simulink model "Vicon_04Sep2012_2Agents"  (Simulink 7.7)
settings: Solver=ode4  StartTime=0.0  StopTime=inf  FixedStep=sample_time  RelTol=1e-3
PreLoadFcn:
  | addpath([cd filesep 'MATLAB_vicon']);
  | addpath([cd filesep 'MATLAB_vicon\Microsoft.VC90.CRT']);
InitFcn:
  | sample_time=0.01;
libraries: simulink x6
settings Model: Creator=ttcl3  LastModifiedBy=Soon Hooi Chiew
settings SolverCC: MaxConsecutiveMinStep=auto
settings DebuggingCC: MultiTaskRateTransMsg=warning

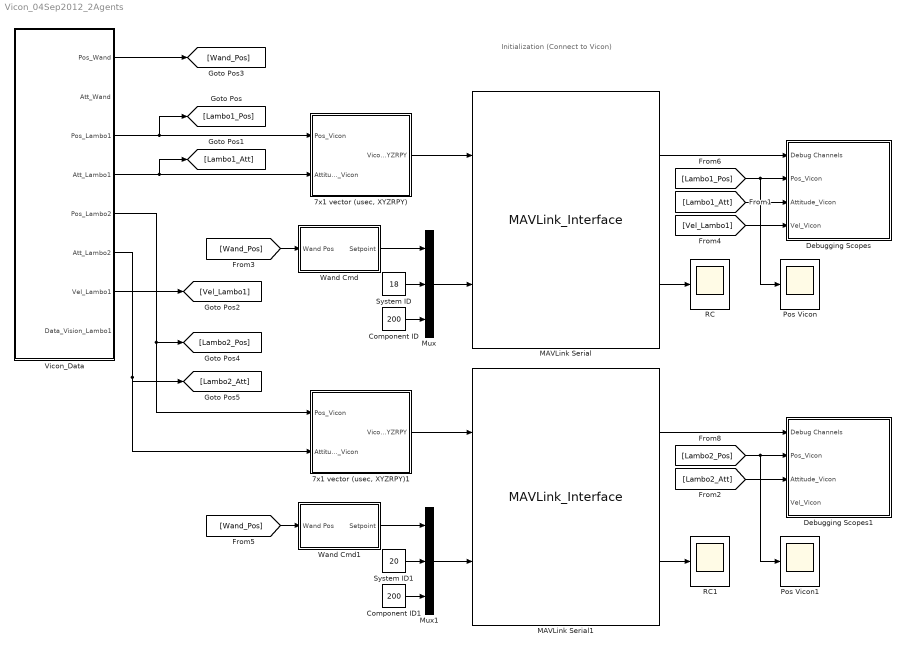
== system Vicon_04Sep2012_2Agents ==
  note: Initialization
      | (Connect to Vicon)
  "7x1 vector (usec, XYZRPY)" : Subsystem
  "7x1 vector (usec, XYZRPY)1" : Subsystem
  Component ID : Constant  Value=200  SampleTime=sample_time
  Component ID1 : Constant  Value=200  SampleTime=sample_time
  Debugging Scopes : Subsystem
  Debugging Scopes1 : Subsystem
  MAVLink Serial : S-Function  FunctionName=MAVLink_Interface  Parameters=COM_Port,Baud_Rate,MSG_INPUT,MSG_OUTPUT  EnableBusSupport=off  mask{COM_Port='COM8', Baud_Rate=57600, HEART_BEAT=off, ATTITUDE_OUT=on, RAW_IMU=off, POSITION_OUT=off, VFR_HUD=off, RC_SCALED=on, SERVO_OUT_RAW=off, VICON_XYZ_RPY_Output=off, SET_MODE=off, DATA_STREAM=off, ATTITUDE_COMMAND=off, ATTITUDE_IN=off, GPS_RAW_IN=off, VFR_HUD_IN=off, VICON_XYZ_RPY=on, VICON_VEL=off, POSITION_DESIRED=on}
      mask prompts: COM_Port "COM Port"; Baud_Rate "Baud Rate"; HEART_BEAT "HEART BEAT"; ATTITUDE_OUT "ATTITUDE"; RAW_IMU "RAW IMU"; POSITION_OUT "GLOBAL POSITION"; VFR_HUD "VFR HUD"; RC_SCALED "RC CHANNELS SCALED"; SERVO_OUT_RAW "SERVO OUTPUT RAW"; VICON_XYZ_RPY_Output "VICON Output"; SET_MODE "SET MODE"; DATA_STREAM "REQUEST DATA STREAM"; ATTITUDE_COMMAND "ATTITUDE COMMAND"; ATTITUDE_IN "ATTITUDE (HIL)"; GPS_RAW_IN "GPS RAW (HIL)"; VFR_HUD_IN "AIRSPEED (HIL)"; VICON_XYZ_RPY "VICON POSITION"; VICON_VEL "VICON SPEED"; POSITION_DESIRED "Position Desired"
      mask init:
      | MSG_ID_NUM_INPUT = [uint8(11) uint8(66) uint8(59) uint8(30) uint8(32) uint8(73) uint8(104) uint8(103) uint8(50)];
      | MSG_ID_NAME_INPUT = [SET_MODE DATA_STREAM ATTITUDE_COMMAND ATTITUDE_IN GPS_RAW_IN VFR_HUD_IN VICON_XYZ_RPY VICON_VEL POSITION_DESIRED];
      | 
      | MSG_ID_NUM_OUTPUT = [uint8(0) uint8(30) uint8(27) uint8(73) uint8(74) uint8(34) uint8(37) uint8(104)];
      | MSG_ID_NAME_OUTPUT = [HEART_BEAT ATTITUDE_OUT RAW_IMU VFR_HUD POSITION_OUT RC_SCALED SERVO_OUT_RAW VICON_XYZ_RPY_Output];
      | 
      | idx_input = find(MSG_ID_NAME_INPUT);
      | MSG_INPUT = MSG_ID_NUM_INPUT(idx_input);
      | 
      | idx_output = find(MSG_ID_NAME_OUTPUT);
      | MSG_OUTPUT = MSG_ID_NUM_OUTPUT(idx_output);
      mask TabNameString: Setting,Setting,Output Message,Output Message,Output Message,Output Message,Output Message,Output Message,Output Message,Output Message,Input Message,Input Message,Input Message,Input Message,Input Message,Input Message,Input Message,Input Message,Input Message
      mask Display:
      | %Label block
      | fprintf('MAVLink Serial\n%s\n%dbps', COM_Port,  Baud_Rate)
      | 
      | %Label input ports
      | 
      | in = 1;
      | if (SET_MODE == 1)
      |     port_label('input', in, 'SET MODE');
      |     in = in + 1;
      | end
      | if (DATA_STREAM == 1)
      |     port_label('input', in, 'REQUEST DATA STREAM');
      |     in = in + 1;
      | end
      | if (ATTITUDE_COMMAND == 1)
      |     port_label('input', in, 'ATTITUDE COMMAND');
      |     in = in + 1;
      | end
      | if (ATTITUDE_IN == 1)
      |     port_label('input', in, 'ATTITUDE (HIL)');
      |     in = in + 1;
      | end
      | if (GPS_RAW_IN == 1)
      |     port_label('input', in, 'GPS RAW (HIL)');
      |     in = in + 1;
      | end
      | if (VFR_HUD_IN == 1)
      |     port_label('input', in, 'AIRSPEED (HIL)');
      |     in = in + 1;
      | end
      | if (VICON_XYZ_RPY == 1)
      |     port_label('input', in, 'VICON XYZ RPY');
      |     in = in + 1;
      | end
      | if (VICON_VEL == 1)
      |     port_label('input', in, 'VICON_VEL');
      |     in = in + 1;
      | end
      | 
      | if (POSITION_DESIRED == 1)
      |     port_label('input', in, 'POSITION_DESIRED');
      |     in = in + 1;
      | end
      | 
      | %Label output ports
      | 
      | out = 1;
      | if (HEART_BEAT == 1)
      |     port_label('output', out, 'HEART BEAT');
      |     out = out + 1;
      | end
      | if (ATTITUDE_OUT == 1)
      |     port_label('output', out, 'ATTITUDE');
      |     out = out + 1;
      | end
      | if (RAW_IMU == 1)
      |     port_label('output', out, 'RAW IMU');
      |     out = out + 1;
      | end
      | if (POSITION_OUT == 1)
      |     port_label('output', out, 'GLOBAL POSITION');
      |     out = out + 1;
      | end
      | if (VFR_HUD == 1)
      |     port_label('output', out, 'VFR HUD');
      |     out = out + 1;
      | end
      | if (RC_SCALED == 1)
      |     port_label('output', out, 'RC CHANNELS SCALED');
      |     out = out + 1;
      | end
      | if (SERVO_OUT_RAW == 1)
      |     port_label('output', out, 'SERVO OUTPUT RAW');
      |     out = out + 1;
      | end
      | % weihua, vicon output
      | if (VICON_XYZ_RPY_Output == 1)
      |     port_label('output', out, 'VICON_XYZ_RPY');
      |     out = out + 1;
      | end
  MAVLink Serial1 : S-Function  FunctionName=MAVLink_Interface  Parameters=COM_Port,Baud_Rate,MSG_INPUT,MSG_OUTPUT  EnableBusSupport=off  mask{COM_Port='COM4', Baud_Rate=57600, HEART_BEAT=off, ATTITUDE_OUT=on, RAW_IMU=off, POSITION_OUT=off, VFR_HUD=off, RC_SCALED=on, SERVO_OUT_RAW=off, VICON_XYZ_RPY_Output=off, SET_MODE=off, DATA_STREAM=off, ATTITUDE_COMMAND=off, ATTITUDE_IN=off, GPS_RAW_IN=off, VFR_HUD_IN=off, VICON_XYZ_RPY=on, VICON_VEL=off, POSITION_DESIRED=on}
      mask prompts: COM_Port "COM Port"; Baud_Rate "Baud Rate"; HEART_BEAT "HEART BEAT"; ATTITUDE_OUT "ATTITUDE"; RAW_IMU "RAW IMU"; POSITION_OUT "GLOBAL POSITION"; VFR_HUD "VFR HUD"; RC_SCALED "RC CHANNELS SCALED"; SERVO_OUT_RAW "SERVO OUTPUT RAW"; VICON_XYZ_RPY_Output "VICON Output"; SET_MODE "SET MODE"; DATA_STREAM "REQUEST DATA STREAM"; ATTITUDE_COMMAND "ATTITUDE COMMAND"; ATTITUDE_IN "ATTITUDE (HIL)"; GPS_RAW_IN "GPS RAW (HIL)"; VFR_HUD_IN "AIRSPEED (HIL)"; VICON_XYZ_RPY "VICON POSITION"; VICON_VEL "VICON SPEED"; POSITION_DESIRED "Position Desired"
      mask init: same as Vicon_04Sep2012_2Agents/MAVLink Serial
      mask TabNameString: Setting,Setting,Output Message,Output Message,Output Message,Output Message,Output Message,Output Message,Output Message,Output Message,Input Message,Input Message,Input Message,Input Message,Input Message,Input Message,Input Message,Input Message,Input Message
      mask Display:
      | %Label block
      | fprintf('MAVLink Serial\n%s\n%dbps', COM_Port,  Baud_Rate)
      | 
      | %Label input ports
      | 
      | in = 1;
      | if (SET_MODE == 1)
      |     port_label('input', in, 'SET MODE');
      |     in = in + 1;
      | end
      | if (DATA_STREAM == 1)
      |     port_label('input', in, 'REQUEST DATA STREAM');
      |     in = in + 1;
      | end
      | if (ATTITUDE_COMMAND == 1)
      |     port_label('input', in, 'ATTITUDE COMMAND');
      |     in = in + 1;
      | end
      | if (ATTITUDE_IN == 1)
      |     port_label('input', in, 'ATTITUDE (HIL)');
      |     in = in + 1;
      | end
      | if (GPS_RAW_IN == 1)
      |     port_label('input', in, 'GPS RAW (HIL)');
      |     in = in + 1;
      | end
      | if (VFR_HUD_IN == 1)
      |     port_label('input', in, 'AIRSPEED (HIL)');
      |     in = in + 1;
      | end
      | if (VICON_XYZ_RPY == 1)
      |     port_label('input', in, 'VICON XYZ RPY');
      |     in = in + 1;
      | end
      | if (VICON_VEL == 1)
      |     port_label('input', in, 'VICON_VEL');
      |     in = in + 1;
      | end
      | 
      | if (POSITION_DESIRED == 1)
      |     port_label('input', in, 'POSITION_DESIRED');
      |     in = in + 1;
      | end
      | 
      | %Label output ports
      | 
      | out = 1;
      | if (HEART_BEAT == 1)
      |     port_label('output', out, 'HEART BEAT');
      |     out = out + 1;
      | end
      | if (ATTITUDE_OUT == 1)
      |     port_label('output', out, 'ATTITUDE');
      |     out = out + 1;
      | end
      | if (RAW_IMU == 1)
      |     port_label('output', out, 'RAW IMU');
      |     out = out + 1;
      | end
      | if (POSITION_OUT == 1)
      |     port_label('output', out, 'GLOBAL POSITION');
      |     out = out + 1;
      | end
      | if (VFR_HUD == 1)
      |     port_label('output', out, 'VFR HUD');
      |     out = out + 1;
      | end
      | if (RC_SCALED == 1)
      |     port_label('output', out, 'RC CHANNELS SCALED');
      |     out = out + 1;
      | end
      | if (SERVO_OUT_RAW == 1)
      |     port_label('output', out, 'SERVO OUTPUT RAW');
      |     out = out + 1;
      | end
      | % weihua, vicon output
      | if (VICON_XYZ_RPY_Output == 1)
      |     port_label('output', out, 'VICON_XYZ_RPY');
      |     out = out + 1;
      | end
  Mux : Mux  Inputs=3
  Mux1 : Mux  Inputs=3
  Pos Vicon : Scope
      settings: TickLabels=on  TimeRange=30  YMin=-3  YMax=3.5  SaveName=ScopeData3  SampleInput=on
  Pos Vicon1 : Scope
      settings: TickLabels=on  TimeRange=30  YMin=-3  YMax=3.5  SaveName=ScopeData17  SampleInput=on
  RC : Scope
      settings: TickLabels=on  TimeRange=30  YMin=-1  YMax=0.1  SaveName=ScopeData2  SampleInput=on
  RC1 : Scope
      settings: TickLabels=on  TimeRange=30  YMin=-1  YMax=0.1  SaveName=ScopeData18  SampleInput=on
  System ID : Constant  Value=18  SampleTime=sample_time
  System ID1 : Constant  Value=20  SampleTime=sample_time
  Vicon_Data : Subsystem
  Wand Cmd : Subsystem
  Wand Cmd1 : Subsystem
  wires:
  MAVLink Serial/1 -> Debugging Scopes/1(Debug Channels)
  [Lambo1_Pos] -> Debugging Scopes/2(Pos_Vicon), Pos Vicon/1
  [Lambo1_Att] -> Debugging Scopes/3(Attitude_Vicon)
  "7x1 vector (usec, XYZRPY)"/1(Vicon XYZRPY) -> MAVLink Serial/1
  Vicon_Data/4(Att_Lambo1) -> [Lambo1_Att], "7x1 vector (usec, XYZRPY)"/2(Attitude_Vicon)
  Mux/1 -> MAVLink Serial/2
  System ID/1 -> Mux/2
  Component ID/1 -> Mux/3
  [Vel_Lambo1] -> Debugging Scopes/4(Vel_Vicon)
  Vicon_Data/7(Vel_Lambo1) -> [Vel_Lambo1]
  Vicon_Data/3(Pos_Lambo1) -> "7x1 vector (usec, XYZRPY)"/1(Pos_Vicon), [Lambo1_Pos]
  Wand Cmd/1(Setpoint) -> Mux/1
  [Wand_Pos] -> Wand Cmd/1(Wand Pos)
  Vicon_Data/1(Pos_Wand) -> [Wand_Pos]
  MAVLink Serial/2 -> RC/1
  MAVLink Serial1/1 -> Debugging Scopes1/1(Debug Channels)
  [Lambo2_Pos] -> Pos Vicon1/1, Debugging Scopes1/2(Pos_Vicon)
  [Lambo2_Att] -> Debugging Scopes1/3(Attitude_Vicon)
  "7x1 vector (usec, XYZRPY)1"/1(Vicon XYZRPY) -> MAVLink Serial1/1
  Mux1/1 -> MAVLink Serial1/2
  System ID1/1 -> Mux1/2
  Component ID1/1 -> Mux1/3
  Wand Cmd1/1(Setpoint) -> Mux1/1
  [Wand_Pos] -> Wand Cmd1/1(Wand Pos)
  MAVLink Serial1/2 -> RC1/1
  Vicon_Data/5(Pos_Lambo2) -> "7x1 vector (usec, XYZRPY)1"/1(Pos_Vicon), [Lambo2_Pos]
  Vicon_Data/6(Att_Lambo2) -> "7x1 vector (usec, XYZRPY)1"/2(Attitude_Vicon), [Lambo2_Att]

== system Vicon_04Sep2012_2Agents/7x1 vector (usec, XYZRPY) ==
  Pos_Vicon : Inport
  Attitude_Vicon : Inport  Port=2
  Mux1 : Mux  Inputs=3
  usec : Constant  Value=0
  Vicon XYZRPY : Outport
  wires:
  usec/1 -> Mux1/1
  Pos_Vicon/1 -> Mux1/2
  Attitude_Vicon/1 -> Mux1/3
  Mux1/1 -> Vicon XYZRPY/1

== system Vicon_04Sep2012_2Agents/7x1 vector (usec, XYZRPY)1 ==
  Pos_Vicon : Inport
  Attitude_Vicon : Inport  Port=2
  Mux1 : Mux  Inputs=3
  usec : Constant  Value=0
  Vicon XYZRPY : Outport
  wires:
  Mux1/1 -> Vicon XYZRPY/1
  Attitude_Vicon/1 -> Mux1/3
  Pos_Vicon/1 -> Mux1/2
  usec/1 -> Mux1/1

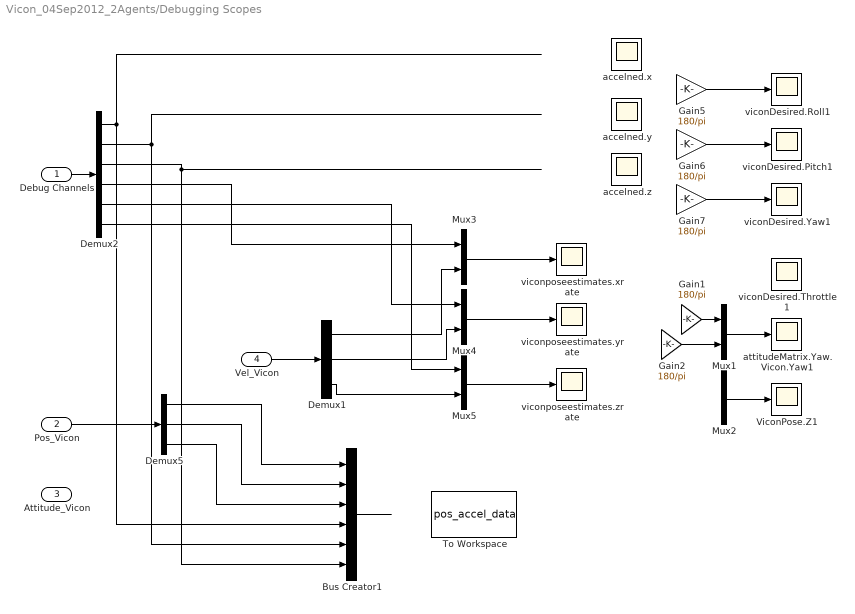
== system Vicon_04Sep2012_2Agents/Debugging Scopes ==
  Debug Channels : Inport
  Pos_Vicon : Inport  Port=2
  Attitude_Vicon : Inport  Port=3
  Vel_Vicon : Inport  Port=4
  Bus Creator1 : BusCreator  Inputs=6
  Demux1 : Demux  Outputs=3
  Demux2 : Demux  Outputs=6
  Demux5 : Demux  Outputs=3
  Gain{1..2,5..7} (5 alike) : Gain  Gain=180/pi
  Mux{1..5} (5 alike) : Mux  Inputs=2
  To Workspace : ToWorkspace  VariableName=pos_accel_data  SampleTime=sample_time  SaveFormat=Structure With Time
  ViconPose.Z1 : Scope
      settings: TickLabels=on  TimeRange=60  YMin=-0.475  YMax=-0.2  SaveName=ScopeData9  SampleInput=on
  accelned.x : Scope
      settings: TickLabels=on  TimeRange=60  YMin=-0.06  YMax=-0.0325  SampleInput=on
  accelned.y : Scope
      settings: TickLabels=on  TimeRange=25  YMin=4.12  YMax=4.34  SaveName=ScopeData13  SampleInput=on
  accelned.z : Scope
      settings: TickLabels=on  TimeRange=60  YMin=0.18  YMax=0.31  SaveName=ScopeData14  SampleInput=on
  attitudeMatrix.Yaw. Vicon.Yaw1 : Scope
      settings: TickLabels=on  TimeRange=60  YMin=-81  YMax=-72.5  SaveName=ScopeData15  SampleInput=on
  viconDesired.Pitch1 : Scope
      settings: TickLabels=on  TimeRange=25  YMin=-10.5  YMax=1  SaveName=ScopeData6  SampleInput=on
  viconDesired.Roll1 : Scope
      settings: TickLabels=on  TimeRange=60  YMax=7  SaveName=ScopeData7  SampleInput=on
  viconDesired.Throttle1 : Scope
      settings: TickLabels=on  TimeRange=60  YMin=0  YMax=0.5  SaveName=ScopeData16  SampleInput=on
  viconDesired.Yaw1 : Scope
      settings: TickLabels=on  TimeRange=60  YMin=-0.125  YMax=-0.0725  SaveName=ScopeData8  SampleInput=on
  viconposeestimates.xrate : Scope
      settings: TickLabels=on  TimeRange=60  YMin=-0.0175  YMax=0.0175  SampleInput=on
  viconposeestimates.yrate : Scope
      settings: TickLabels=on  TimeRange=60  YMin=-0.015  YMax=0.0125  SaveName=ScopeData11  SampleInput=on
  viconposeestimates.zrate : Scope
      settings: TickLabels=on  TimeRange=60  YMin=-10  YMax=60  SaveName=ScopeData12  SampleInput=on
  wires:
  Demux2/1 -> Bus Creator1/4
  Demux2/2 -> Bus Creator1/5
  Demux2/3 -> Bus Creator1/6
  Demux5/3 -> Bus Creator1/3
  Demux5/1 -> Bus Creator1/1
  Demux5/2 -> Bus Creator1/2
  Bus Creator1/1 -> ?
  Debug Channels/1 -> Demux2/1
  Pos_Vicon/1 -> Demux5/1
  Gain5/1 -> viconDesired.Roll1/1
  Gain6/1 -> viconDesired.Pitch1/1
  Gain7/1 -> viconDesired.Yaw1/1
  Mux1/1 -> attitudeMatrix.Yaw. Vicon.Yaw1/1
  Mux2/1 -> ViconPose.Z1/1
  Gain1/1 -> Mux1/1
  Gain2/1 -> Mux1/2
  Vel_Vicon/1 -> Demux1/1
  Demux2/4 -> Mux3/1
  Demux2/5 -> Mux4/1
  Demux2/6 -> Mux5/1
  Demux1/3 -> Mux5/2
  Mux3/1 -> viconposeestimates.xrate/1
  Mux4/1 -> viconposeestimates.yrate/1
  Mux5/1 -> viconposeestimates.zrate/1
  Demux1/1 -> Mux3/2
  Demux1/2 -> Mux4/2

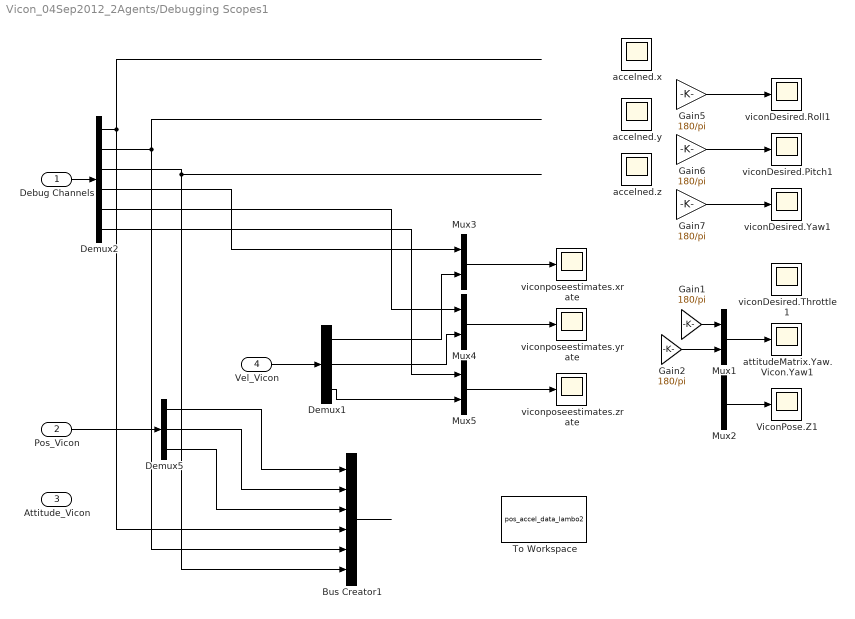
== system Vicon_04Sep2012_2Agents/Debugging Scopes1 ==
  Debug Channels : Inport
  Pos_Vicon : Inport  Port=2
  Attitude_Vicon : Inport  Port=3
  Vel_Vicon : Inport  Port=4
  Bus Creator1 : BusCreator  Inputs=6
  Demux1 : Demux  Outputs=3
  Demux2 : Demux  Outputs=6
  Demux5 : Demux  Outputs=3
  Gain{1..2,5..7} (5 alike) : Gain  Gain=180/pi
  Mux{1..5} (5 alike) : Mux  Inputs=2
  To Workspace : ToWorkspace  VariableName=pos_accel_data_lambo2  SampleTime=sample_time  SaveFormat=Structure With Time
  ViconPose.Z1 : Scope
      settings: TickLabels=on  TimeRange=60  YMin=-0.475  YMax=-0.2  SaveName=ScopeData9  SampleInput=on
  accelned.x : Scope
      settings: TickLabels=on  TimeRange=60  YMin=-0.06  YMax=-0.0325  SampleInput=on
  accelned.y : Scope
      settings: TickLabels=on  TimeRange=25  YMin=4.12  YMax=4.34  SaveName=ScopeData13  SampleInput=on
  accelned.z : Scope
      settings: TickLabels=on  TimeRange=60  YMin=0.18  YMax=0.31  SaveName=ScopeData14  SampleInput=on
  attitudeMatrix.Yaw. Vicon.Yaw1 : Scope
      settings: TickLabels=on  TimeRange=60  YMin=-81  YMax=-72.5  SaveName=ScopeData15  SampleInput=on
  viconDesired.Pitch1 : Scope
      settings: TickLabels=on  TimeRange=25  YMin=-10.5  YMax=1  SaveName=ScopeData6  SampleInput=on
  viconDesired.Roll1 : Scope
      settings: TickLabels=on  TimeRange=60  YMax=7  SaveName=ScopeData7  SampleInput=on
  viconDesired.Throttle1 : Scope
      settings: TickLabels=on  TimeRange=60  YMin=0  YMax=0.5  SaveName=ScopeData16  SampleInput=on
  viconDesired.Yaw1 : Scope
      settings: TickLabels=on  TimeRange=60  YMin=-0.125  YMax=-0.0725  SaveName=ScopeData8  SampleInput=on
  viconposeestimates.xrate : Scope
      settings: TickLabels=on  TimeRange=60  YMin=-0.0175  YMax=0.0175  SampleInput=on
  viconposeestimates.yrate : Scope
      settings: TickLabels=on  TimeRange=60  YMin=-0.015  YMax=0.0125  SaveName=ScopeData11  SampleInput=on
  viconposeestimates.zrate : Scope
      settings: TickLabels=on  TimeRange=60  YMin=-10  YMax=60  SaveName=ScopeData12  SampleInput=on
  wires:
  Demux1/2 -> Mux4/2
  Demux1/1 -> Mux3/2
  Mux5/1 -> viconposeestimates.zrate/1
  Mux4/1 -> viconposeestimates.yrate/1
  Mux3/1 -> viconposeestimates.xrate/1
  Demux1/3 -> Mux5/2
  Demux2/6 -> Mux5/1
  Demux2/5 -> Mux4/1
  Demux2/4 -> Mux3/1
  Vel_Vicon/1 -> Demux1/1
  Gain2/1 -> Mux1/2
  Gain1/1 -> Mux1/1
  Mux2/1 -> ViconPose.Z1/1
  Mux1/1 -> attitudeMatrix.Yaw. Vicon.Yaw1/1
  Gain7/1 -> viconDesired.Yaw1/1
  Gain6/1 -> viconDesired.Pitch1/1
  Gain5/1 -> viconDesired.Roll1/1
  Pos_Vicon/1 -> Demux5/1
  Debug Channels/1 -> Demux2/1
  Bus Creator1/1 -> ?
  Demux5/2 -> Bus Creator1/2
  Demux5/1 -> Bus Creator1/1
  Demux5/3 -> Bus Creator1/3
  Demux2/3 -> Bus Creator1/6
  Demux2/2 -> Bus Creator1/5
  Demux2/1 -> Bus Creator1/4

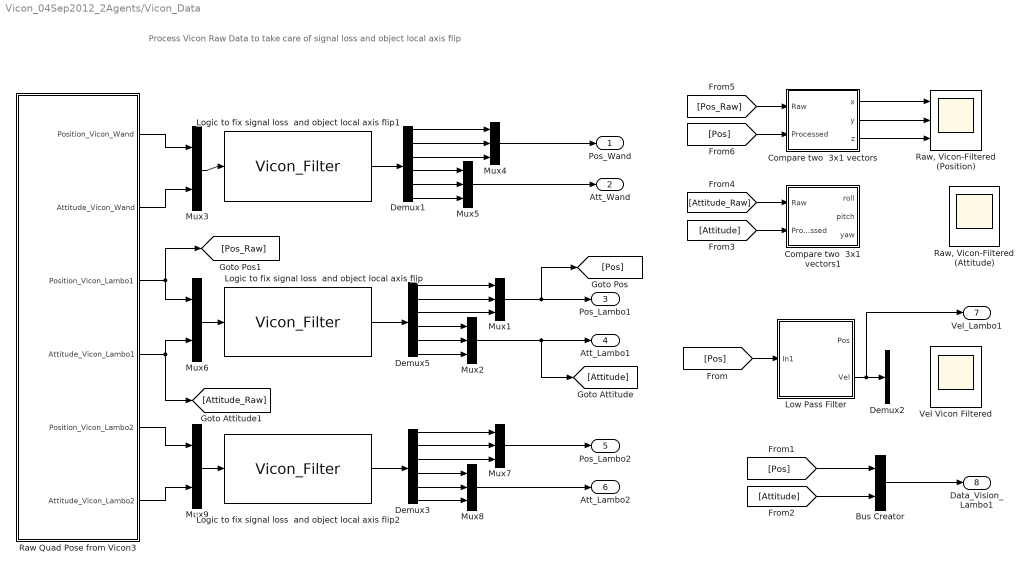
== system Vicon_04Sep2012_2Agents/Vicon_Data ==
  note: Process Vicon Raw Data to take care of signal loss and object local axis flip
  Bus Creator : BusCreator  Inputs=2
  Compare two  3x1 vectors : Subsystem
  Compare two  3x1 vectors1 : Subsystem
  Demux1 : Demux  Outputs=6
  Demux2 : Demux  Outputs=3
  Demux3 : Demux  Outputs=6
  Demux5 : Demux  Outputs=6
  Logic to fix signal loss  and object local axis flip : M-S-Function  FunctionName=Vicon_Filter
  Logic to fix signal loss  and object local axis flip1 : M-S-Function  FunctionName=Vicon_Filter
  Logic to fix signal loss  and object local axis flip2 : M-S-Function  FunctionName=Vicon_Filter
  Low Pass Filter : Subsystem
  Mux{1..2,4..5,7..8} (6 alike) : Mux  Inputs=3
  Mux3 : Mux  Inputs=2
  Mux6 : Mux  Inputs=2
  Mux9 : Mux  Inputs=2
  Raw Quad Pose from Vicon3 : Subsystem
  "Raw, Vicon-Filtered (Attitude)" : Scope  NumInputPorts=3
      settings: TimeRange=50  YMin=-3.14159~-1~-3.5  YMax=3.14159~1~3.5  SaveName=ScopeData4
  "Raw, Vicon-Filtered (Position)" : Scope  NumInputPorts=3
      settings: TimeRange=50  YMin=-2.09~2.281~-0.0655  YMax=-2.055~2.293~-0.063  SaveName=ScopeData10
  "Vel Vicon Filtered " : Scope  NumInputPorts=3
      settings: YMin=-0.7~-1~-9  YMax=0.4~7.5~0.5  SaveName=ScopeData5
  Pos_Wand : Outport
  Att_Wand : Outport  Port=2
  Pos_Lambo1 : Outport  Port=3
  Att_Lambo1 : Outport  Port=4
  Pos_Lambo2 : Outport  Port=5
  Att_Lambo2 : Outport  Port=6
  Vel_Lambo1 : Outport  Port=7
  Data_Vision_Lambo1 : Outport  Port=8
  wires:
  Compare two  3x1 vectors/1(x) -> "Raw, Vicon-Filtered (Position)"/1
  Compare two  3x1 vectors/2(y) -> "Raw, Vicon-Filtered (Position)"/2
  Low Pass Filter/2(Vel) -> Demux2/1, Vel_Lambo1/1
  Logic to fix signal loss  and object local axis flip/1 -> Demux5/1
  Demux5/1 -> Mux1/1
  Demux5/2 -> Mux1/2
  Demux5/3 -> Mux1/3
  Demux5/4 -> Mux2/1
  Demux5/5 -> Mux2/2
  Demux5/6 -> Mux2/3
  Mux2/1 -> Att_Lambo1/1, [Attitude]
  [Pos] -> Low Pass Filter/1(In1)
  Compare two  3x1 vectors/3(z) -> "Raw, Vicon-Filtered (Position)"/3
  Mux1/1 -> Pos_Lambo1/1, [Pos]
  [Attitude_Raw] -> Compare two  3x1 vectors1/1(Raw)
  [Attitude] -> Compare two  3x1 vectors1/2(Processed)
  [Pos_Raw] -> Compare two  3x1 vectors/1(Raw)
  [Pos] -> Compare two  3x1 vectors/2(Processed)
  [Pos] -> Bus Creator/1
  [Attitude] -> Bus Creator/2
  Bus Creator/1 -> Data_Vision_Lambo1/1
  Mux3/1 -> Logic to fix signal loss  and object local axis flip1/1
  Logic to fix signal loss  and object local axis flip1/1 -> Demux1/1
  Demux1/1 -> Mux4/1
  Demux1/2 -> Mux4/2
  Demux1/3 -> Mux4/3
  Demux1/4 -> Mux5/1
  Demux1/5 -> Mux5/2
  Demux1/6 -> Mux5/3
  Mux5/1 -> Att_Wand/1
  Mux4/1 -> Pos_Wand/1
  Raw Quad Pose from Vicon3/1(Position_Vicon_Wand) -> Mux3/1
  Raw Quad Pose from Vicon3/2(Attitude_Vicon_Wand) -> Mux3/2
  Raw Quad Pose from Vicon3/3(Position_Vicon_Lambo1) -> Mux6/1, [Pos_Raw]
  Raw Quad Pose from Vicon3/4(Attitude_Vicon_Lambo1) -> Mux6/2, [Attitude_Raw]
  Mux6/1 -> Logic to fix signal loss  and object local axis flip/1
  Logic to fix signal loss  and object local axis flip2/1 -> Demux3/1
  Demux3/1 -> Mux7/1
  Demux3/2 -> Mux7/2
  Demux3/3 -> Mux7/3
  Demux3/4 -> Mux8/1
  Demux3/5 -> Mux8/2
  Demux3/6 -> Mux8/3
  Mux8/1 -> Att_Lambo2/1
  Mux7/1 -> Pos_Lambo2/1
  Mux9/1 -> Logic to fix signal loss  and object local axis flip2/1
  Raw Quad Pose from Vicon3/5(Position_Vicon_Lambo2) -> Mux9/1
  Raw Quad Pose from Vicon3/6(Attitude_Vicon_Lambo2) -> Mux9/2

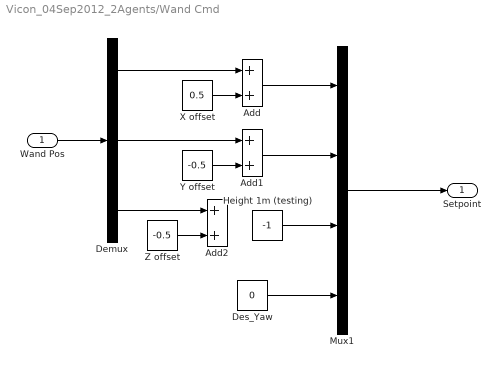
== system Vicon_04Sep2012_2Agents/Wand Cmd ==
  Wand Pos : Inport
  Add : Sum
  Add1 : Sum
  Add2 : Sum
  Demux : Demux  Outputs=3
  Des_Yaw : Constant  Value=0  SampleTime=sample_time
  Height 1m (testing) : Constant  Value=-1  SampleTime=sample_time
  Mux1 : Mux
  X offset : Constant  Value=0.5
  Y offset : Constant  Value=-0.5
  Z offset : Constant  Value=-0.5
  Setpoint : Outport
  wires:
  Wand Pos/1 -> Demux/1
  Mux1/1 -> Setpoint/1
  Demux/1 -> Add/1
  X offset/1 -> Add/2
  Demux/2 -> Add1/1
  Y offset/1 -> Add1/2
  Demux/3 -> Add2/1
  Z offset/1 -> Add2/2
  Add/1 -> Mux1/1
  Add1/1 -> Mux1/2
  Des_Yaw/1 -> Mux1/4
  Height 1m (testing)/1 -> Mux1/3

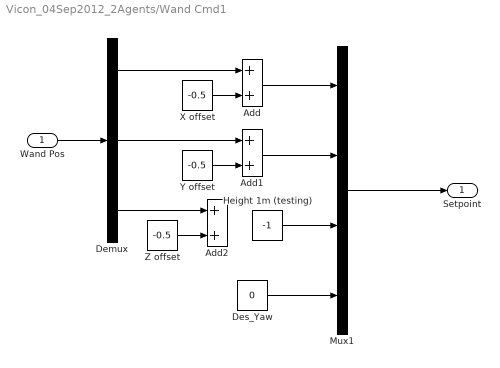
== system Vicon_04Sep2012_2Agents/Wand Cmd1 ==
  Wand Pos : Inport
  Add : Sum
  Add1 : Sum
  Add2 : Sum
  Demux : Demux  Outputs=3
  Des_Yaw : Constant  Value=0  SampleTime=sample_time
  Height 1m (testing) : Constant  Value=-1  SampleTime=sample_time
  Mux1 : Mux
  X offset : Constant  Value=-0.5
  Y offset : Constant  Value=-0.5
  Z offset : Constant  Value=-0.5
  Setpoint : Outport
  wires:
  Height 1m (testing)/1 -> Mux1/3
  Des_Yaw/1 -> Mux1/4
  Add1/1 -> Mux1/2
  Add/1 -> Mux1/1
  Z offset/1 -> Add2/2
  Demux/3 -> Add2/1
  Y offset/1 -> Add1/2
  Demux/2 -> Add1/1
  X offset/1 -> Add/2
  Demux/1 -> Add/1
  Mux1/1 -> Setpoint/1
  Wand Pos/1 -> Demux/1

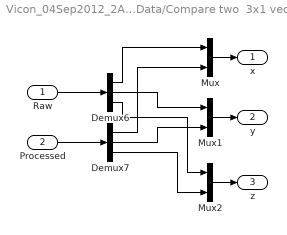
== system Vicon_04Sep2012_2Agents/Vicon_Data/Compare two  3x1 vectors ==
  Raw : Inport
  Processed : Inport  Port=2
  Demux6 : Demux  Outputs=3
  Demux7 : Demux  Outputs=3
  Mux : Mux  Inputs=2
  Mux1 : Mux  Inputs=2
  Mux2 : Mux  Inputs=2
  x : Outport
  y : Outport  Port=2
  z : Outport  Port=3
  wires:
  Demux6/1 -> Mux/1
  Demux6/2 -> Mux1/1
  Demux7/2 -> Mux1/2
  Demux6/3 -> Mux2/1
  Demux7/3 -> Mux2/2
  Raw/1 -> Demux6/1
  Processed/1 -> Demux7/1
  Mux/1 -> x/1
  Mux1/1 -> y/1
  Mux2/1 -> z/1
  Demux7/1 -> Mux/2

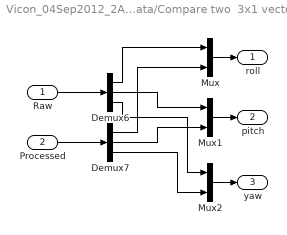
== system Vicon_04Sep2012_2Agents/Vicon_Data/Compare two  3x1 vectors1 ==
  Raw : Inport
  Processed : Inport  Port=2
  Demux6 : Demux  Outputs=3
  Demux7 : Demux  Outputs=3
  Mux : Mux  Inputs=2
  Mux1 : Mux  Inputs=2
  Mux2 : Mux  Inputs=2
  roll : Outport
  pitch : Outport  Port=2
  yaw : Outport  Port=3
  wires:
  Demux7/1 -> Mux/2
  Mux2/1 -> yaw/1
  Mux1/1 -> pitch/1
  Mux/1 -> roll/1
  Processed/1 -> Demux7/1
  Raw/1 -> Demux6/1
  Demux7/3 -> Mux2/2
  Demux6/3 -> Mux2/1
  Demux7/2 -> Mux1/2
  Demux6/2 -> Mux1/1
  Demux6/1 -> Mux/1

== system Vicon_04Sep2012_2Agents/Vicon_Data/Low Pass Filter ==
  In1 : Inport
  Gain : Gain  Gain=1/0.01
  Gain1 : Gain  Gain=1/0.1
  Integrator : Integrator
  Integrator1 : Integrator
  Sum : Sum  Inputs=|+-
  Sum1 : Sum  Inputs=|+-
  Pos : Outport
  Vel : Outport  Port=2
  wires:
  Sum/1 -> Gain/1
  Gain/1 -> Integrator/1, Sum1/1, Vel/1
  Integrator/1 -> Pos/1, Sum/2
  In1/1 -> Sum/1
  Sum1/1 -> Gain1/1
  Gain1/1 -> Integrator1/1
  Integrator1/1 -> Sum1/2

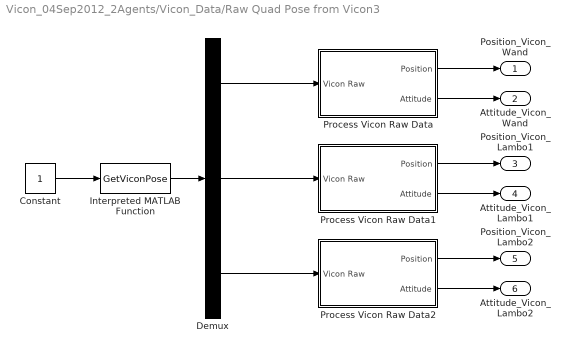
== system Vicon_04Sep2012_2Agents/Vicon_Data/Raw Quad Pose from Vicon3 ==
  Constant : Constant
  Demux : Demux  Outputs=3
  Interpreted MATLAB Function : MATLABFcn  MATLABFcn=GetViconPose
  Process Vicon Raw Data : Subsystem
  Process Vicon Raw Data1 : Subsystem
  Process Vicon Raw Data2 : Subsystem
  Position_Vicon_Wand : Outport
  Attitude_Vicon_Wand : Outport  Port=2
  Position_Vicon_Lambo1 : Outport  Port=3
  Attitude_Vicon_Lambo1 : Outport  Port=4
  Position_Vicon_Lambo2 : Outport  Port=5
  Attitude_Vicon_Lambo2 : Outport  Port=6
  wires:
  Process Vicon Raw Data/2(Attitude) -> Attitude_Vicon_Wand/1
  Process Vicon Raw Data/1(Position) -> Position_Vicon_Wand/1
  Process Vicon Raw Data1/2(Attitude) -> Attitude_Vicon_Lambo1/1
  Process Vicon Raw Data1/1(Position) -> Position_Vicon_Lambo1/1
  Process Vicon Raw Data2/2(Attitude) -> Attitude_Vicon_Lambo2/1
  Process Vicon Raw Data2/1(Position) -> Position_Vicon_Lambo2/1
  Constant/1 -> Interpreted MATLAB Function/1
  Interpreted MATLAB Function/1 -> Demux/1
  Demux/1 -> Process Vicon Raw Data/1(Vicon Raw)
  Demux/2 -> Process Vicon Raw Data1/1(Vicon Raw)
  Demux/3 -> Process Vicon Raw Data2/1(Vicon Raw)

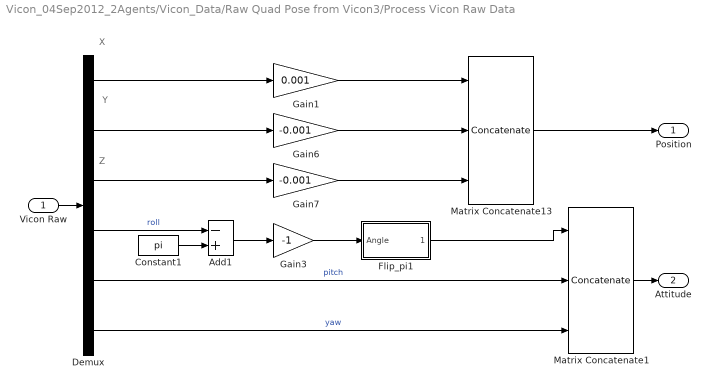
== system Vicon_04Sep2012_2Agents/Vicon_Data/Raw Quad Pose from Vicon3/Process Vicon Raw Data ==
  note: X
  note: Y
  note: Z
  Vicon Raw : Inport
  Add1 : Sum  Inputs=-+
  Constant1 : Constant  Value=pi  OutDataTypeStr=double
  Demux : Demux  Outputs=6
  Flip_pi1 : Subsystem
      mask Type: Flip -pi to pi
      mask Description: Flips the inputs into the range -pi to pi
      mask Help: Flips the inputs into the range -pi to pi
      mask Display: disp('Flip_pi')
  Gain1 : Gain  Gain=0.001
  Gain3 : Gain  Gain=-1
  Gain6 : Gain  Gain=-0.001
  Gain7 : Gain  Gain=-0.001
  Matrix Concatenate1 : Concatenate  NumInputs=3  Mode=Multidimensional array
  Matrix Concatenate13 : Concatenate  NumInputs=3  Mode=Multidimensional array
  Position : Outport
  Attitude : Outport  Port=2
  wires:
  Constant1/1 -> Add1/2
  Demux/6 -> Matrix Concatenate1/3  "yaw"
  Gain1/1 -> Matrix Concatenate13/1
  Demux/1 -> Gain1/1
  Demux/2 -> Gain6/1
  Demux/3 -> Gain7/1
  Demux/4 -> Add1/1  "roll"
  Gain6/1 -> Matrix Concatenate13/2
  Gain7/1 -> Matrix Concatenate13/3
  Add1/1 -> Gain3/1
  Gain3/1 -> Flip_pi1/1(Angle)
  Demux/5 -> Matrix Concatenate1/2  "pitch"
  Flip_pi1/1(Angle_Flip) -> Matrix Concatenate1/1
  Matrix Concatenate13/1 -> Position/1
  Vicon Raw/1 -> Demux/1
  Matrix Concatenate1/1 -> Attitude/1

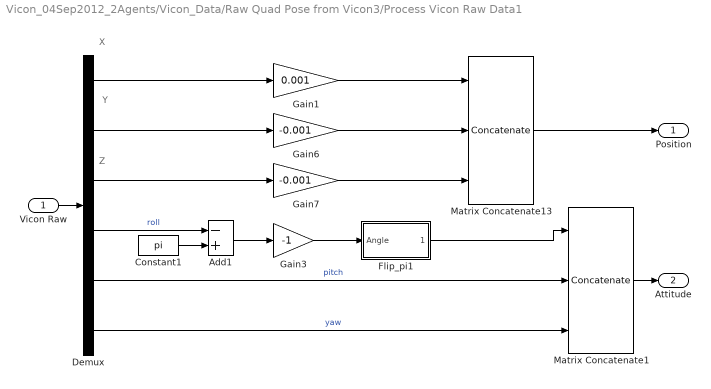
== system Vicon_04Sep2012_2Agents/Vicon_Data/Raw Quad Pose from Vicon3/Process Vicon Raw Data1 ==
  note: Z
  note: Y
  note: X
  Vicon Raw : Inport
  Add1 : Sum  Inputs=-+
  Constant1 : Constant  Value=pi  OutDataTypeStr=double
  Demux : Demux  Outputs=6
  Flip_pi1 : Subsystem
      mask Type: Flip -pi to pi
      mask Description: Flips the inputs into the range -pi to pi
      mask Help: Flips the inputs into the range -pi to pi
      mask Display: disp('Flip_pi')
  Gain1 : Gain  Gain=0.001
  Gain3 : Gain  Gain=-1
  Gain6 : Gain  Gain=-0.001
  Gain7 : Gain  Gain=-0.001
  Matrix Concatenate1 : Concatenate  NumInputs=3  Mode=Multidimensional array
  Matrix Concatenate13 : Concatenate  NumInputs=3  Mode=Multidimensional array
  Position : Outport
  Attitude : Outport  Port=2
  wires:
  Matrix Concatenate1/1 -> Attitude/1
  Vicon Raw/1 -> Demux/1
  Matrix Concatenate13/1 -> Position/1
  Flip_pi1/1(Angle_Flip) -> Matrix Concatenate1/1
  Demux/5 -> Matrix Concatenate1/2  "pitch"
  Gain3/1 -> Flip_pi1/1(Angle)
  Add1/1 -> Gain3/1
  Gain7/1 -> Matrix Concatenate13/3
  Gain6/1 -> Matrix Concatenate13/2
  Demux/4 -> Add1/1  "roll"
  Demux/3 -> Gain7/1
  Demux/2 -> Gain6/1
  Demux/1 -> Gain1/1
  Gain1/1 -> Matrix Concatenate13/1
  Demux/6 -> Matrix Concatenate1/3  "yaw"
  Constant1/1 -> Add1/2

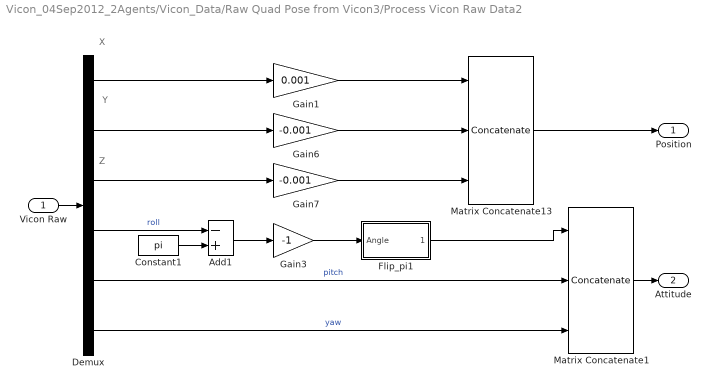
== system Vicon_04Sep2012_2Agents/Vicon_Data/Raw Quad Pose from Vicon3/Process Vicon Raw Data2 ==
  note: X
  note: Y
  note: Z
  Vicon Raw : Inport
  Add1 : Sum  Inputs=-+
  Constant1 : Constant  Value=pi  OutDataTypeStr=double
  Demux : Demux  Outputs=6
  Flip_pi1 : Subsystem
      mask Type: Flip -pi to pi
      mask Description: Flips the inputs into the range -pi to pi
      mask Help: Flips the inputs into the range -pi to pi
      mask Display: disp('Flip_pi')
  Gain1 : Gain  Gain=0.001
  Gain3 : Gain  Gain=-1
  Gain6 : Gain  Gain=-0.001
  Gain7 : Gain  Gain=-0.001
  Matrix Concatenate1 : Concatenate  NumInputs=3  Mode=Multidimensional array
  Matrix Concatenate13 : Concatenate  NumInputs=3  Mode=Multidimensional array
  Position : Outport
  Attitude : Outport  Port=2
  wires:
  Constant1/1 -> Add1/2
  Demux/6 -> Matrix Concatenate1/3  "yaw"
  Gain1/1 -> Matrix Concatenate13/1
  Demux/1 -> Gain1/1
  Demux/2 -> Gain6/1
  Demux/3 -> Gain7/1
  Demux/4 -> Add1/1  "roll"
  Gain6/1 -> Matrix Concatenate13/2
  Gain7/1 -> Matrix Concatenate13/3
  Add1/1 -> Gain3/1
  Gain3/1 -> Flip_pi1/1(Angle)
  Demux/5 -> Matrix Concatenate1/2  "pitch"
  Flip_pi1/1(Angle_Flip) -> Matrix Concatenate1/1
  Matrix Concatenate13/1 -> Position/1
  Vicon Raw/1 -> Demux/1
  Matrix Concatenate1/1 -> Attitude/1

== system Vicon_04Sep2012_2Agents/Vicon_Data/Raw Quad Pose from Vicon3/Process Vicon Raw Data/Flip_pi1 ==
  Angle : Inport
  Add : Sum  Inputs=-+
  Compare To Constant1 : simulink/Logic and Bit Operations/Compare To Constant  SystemSampleTime=-1  relop=>  const=pi  LogicOutDataTypeMode=uint8  ZeroCross=off
  Constant : Constant  Value=2*pi
  Data Type Duplicate : DataTypeDuplicate
  Flip_0_to_2pi : Subsystem
      mask Type: Flip zero to 2pi
      mask Description: Flips the inputs into the range zero to +2pi
      mask Help: Flips the inputs into the range zero to +2pi
      mask Display: disp('Flip_0_2pi')
  Switch : Switch  Criteria=u2 ~= 0
  Angle_Flip : Outport
  wires:
  Switch/1 -> Data Type Duplicate/1, Angle_Flip/1
  Add/1 -> Switch/1
  Constant/1 -> Add/1
  Compare To Constant1/1 -> Switch/2
  Flip_0_to_2pi/1(Angle_Flip) -> Add/2, Compare To Constant1/1, Switch/3
  Angle/1 -> Data Type Duplicate/2, Flip_0_to_2pi/1(Angle)

== system Vicon_04Sep2012_2Agents/Vicon_Data/Raw Quad Pose from Vicon3/Process Vicon Raw Data1/Flip_pi1 ==
  Angle : Inport
  Add : Sum  Inputs=-+
  Compare To Constant1 : simulink/Logic and Bit Operations/Compare To Constant  SystemSampleTime=-1  relop=>  const=pi  LogicOutDataTypeMode=uint8  ZeroCross=off
  Constant : Constant  Value=2*pi
  Data Type Duplicate : DataTypeDuplicate
  Flip_0_to_2pi : Subsystem
      mask Type: Flip zero to 2pi
      mask Description: Flips the inputs into the range zero to +2pi
      mask Help: Flips the inputs into the range zero to +2pi
      mask Display: disp('Flip_0_2pi')
  Switch : Switch  Criteria=u2 ~= 0
  Angle_Flip : Outport
  wires:
  Angle/1 -> Flip_0_to_2pi/1(Angle), Data Type Duplicate/2
  Flip_0_to_2pi/1(Angle_Flip) -> Switch/3, Compare To Constant1/1, Add/2
  Compare To Constant1/1 -> Switch/2
  Constant/1 -> Add/1
  Add/1 -> Switch/1
  Switch/1 -> Angle_Flip/1, Data Type Duplicate/1

== system Vicon_04Sep2012_2Agents/Vicon_Data/Raw Quad Pose from Vicon3/Process Vicon Raw Data2/Flip_pi1 ==
  Angle : Inport
  Add : Sum  Inputs=-+
  Compare To Constant1 : simulink/Logic and Bit Operations/Compare To Constant  SystemSampleTime=-1  relop=>  const=pi  LogicOutDataTypeMode=uint8  ZeroCross=off
  Constant : Constant  Value=2*pi
  Data Type Duplicate : DataTypeDuplicate
  Flip_0_to_2pi : Subsystem
      mask Type: Flip zero to 2pi
      mask Description: Flips the inputs into the range zero to +2pi
      mask Help: Flips the inputs into the range zero to +2pi
      mask Display: disp('Flip_0_2pi')
  Switch : Switch  Criteria=u2 ~= 0
  Angle_Flip : Outport
  wires:
  Switch/1 -> Data Type Duplicate/1, Angle_Flip/1
  Add/1 -> Switch/1
  Constant/1 -> Add/1
  Compare To Constant1/1 -> Switch/2
  Flip_0_to_2pi/1(Angle_Flip) -> Add/2, Compare To Constant1/1, Switch/3
  Angle/1 -> Data Type Duplicate/2, Flip_0_to_2pi/1(Angle)

== system Vicon_04Sep2012_2Agents/Vicon_Data/Raw Quad Pose from Vicon3/Process Vicon Raw Data/Flip_pi1/Flip_0_to_2pi ==
  Angle : Inport
  Add : Sum
  Compare To Constant1 : simulink/Logic and Bit Operations/Compare To Constant  SystemSampleTime=-1  relop=<  const=0  LogicOutDataTypeMode=uint8  ZeroCross=off
  Constant : Constant  Value=2*pi
  Data Type Duplicate : DataTypeDuplicate
  Flip_2pi : Subsystem
      mask Type: Flip -2pi to 2pi
      mask Description: Flips the inputs into the range -2pi to +2pi
      mask Help: Flips the inputs into the range -2pi to +2pi
      mask Display: disp('Flip_2pi')
  Switch : Switch  Criteria=u2 ~= 0
  Angle_Flip : Outport
  wires:
  Switch/1 -> Data Type Duplicate/1, Angle_Flip/1
  Angle/1 -> Data Type Duplicate/2, Flip_2pi/1(Angle)
  Add/1 -> Switch/1
  Constant/1 -> Add/1
  Compare To Constant1/1 -> Switch/2
  Flip_2pi/1(Angle_Flip) -> Switch/3, Add/2, Compare To Constant1/1

== system Vicon_04Sep2012_2Agents/Vicon_Data/Raw Quad Pose from Vicon3/Process Vicon Raw Data1/Flip_pi1/Flip_0_to_2pi ==
  Angle : Inport
  Add : Sum
  Compare To Constant1 : simulink/Logic and Bit Operations/Compare To Constant  SystemSampleTime=-1  relop=<  const=0  LogicOutDataTypeMode=uint8  ZeroCross=off
  Constant : Constant  Value=2*pi
  Data Type Duplicate : DataTypeDuplicate
  Flip_2pi : Subsystem
      mask Type: Flip -2pi to 2pi
      mask Description: Flips the inputs into the range -2pi to +2pi
      mask Help: Flips the inputs into the range -2pi to +2pi
      mask Display: disp('Flip_2pi')
  Switch : Switch  Criteria=u2 ~= 0
  Angle_Flip : Outport
  wires:
  Flip_2pi/1(Angle_Flip) -> Compare To Constant1/1, Add/2, Switch/3
  Compare To Constant1/1 -> Switch/2
  Constant/1 -> Add/1
  Add/1 -> Switch/1
  Angle/1 -> Flip_2pi/1(Angle), Data Type Duplicate/2
  Switch/1 -> Angle_Flip/1, Data Type Duplicate/1

== system Vicon_04Sep2012_2Agents/Vicon_Data/Raw Quad Pose from Vicon3/Process Vicon Raw Data2/Flip_pi1/Flip_0_to_2pi ==
  Angle : Inport
  Add : Sum
  Compare To Constant1 : simulink/Logic and Bit Operations/Compare To Constant  SystemSampleTime=-1  relop=<  const=0  LogicOutDataTypeMode=uint8  ZeroCross=off
  Constant : Constant  Value=2*pi
  Data Type Duplicate : DataTypeDuplicate
  Flip_2pi : Subsystem
      mask Type: Flip -2pi to 2pi
      mask Description: Flips the inputs into the range -2pi to +2pi
      mask Help: Flips the inputs into the range -2pi to +2pi
      mask Display: disp('Flip_2pi')
  Switch : Switch  Criteria=u2 ~= 0
  Angle_Flip : Outport
  wires:
  Switch/1 -> Data Type Duplicate/1, Angle_Flip/1
  Angle/1 -> Data Type Duplicate/2, Flip_2pi/1(Angle)
  Add/1 -> Switch/1
  Constant/1 -> Add/1
  Compare To Constant1/1 -> Switch/2
  Flip_2pi/1(Angle_Flip) -> Switch/3, Add/2, Compare To Constant1/1

== system Vicon_04Sep2012_2Agents/Vicon_Data/Raw Quad Pose from Vicon3/Process Vicon Raw Data/Flip_pi1/Flip_0_to_2pi/Flip_2pi ==
  Angle : Inport
  Bias : Bias  Bias=-2*pi
  Constant : Constant  Value=2*pi
  Data Type Duplicate : DataTypeDuplicate
  Modulo : Math  Operator=mod  SaturateOnIntegerOverflow=on
  Sign1 : Signum
  Switch : Switch
  Angle_Flip : Outport
  wires:
  Switch/1 -> Data Type Duplicate/2, Angle_Flip/1
  Bias/1 -> Switch/3
  Sign1/1 -> Switch/2
  Modulo/1 -> Switch/1, Bias/1
  Constant/1 -> Modulo/2
  Angle/1 -> Data Type Duplicate/1, Sign1/1, Modulo/1

== system Vicon_04Sep2012_2Agents/Vicon_Data/Raw Quad Pose from Vicon3/Process Vicon Raw Data1/Flip_pi1/Flip_0_to_2pi/Flip_2pi ==
  Angle : Inport
  Bias : Bias  Bias=-2*pi
  Constant : Constant  Value=2*pi
  Data Type Duplicate : DataTypeDuplicate
  Modulo : Math  Operator=mod  SaturateOnIntegerOverflow=on
  Sign1 : Signum
  Switch : Switch
  Angle_Flip : Outport
  wires:
  Angle/1 -> Modulo/1, Sign1/1, Data Type Duplicate/1
  Constant/1 -> Modulo/2
  Modulo/1 -> Bias/1, Switch/1
  Sign1/1 -> Switch/2
  Bias/1 -> Switch/3
  Switch/1 -> Angle_Flip/1, Data Type Duplicate/2

== system Vicon_04Sep2012_2Agents/Vicon_Data/Raw Quad Pose from Vicon3/Process Vicon Raw Data2/Flip_pi1/Flip_0_to_2pi/Flip_2pi ==
  Angle : Inport
  Bias : Bias  Bias=-2*pi
  Constant : Constant  Value=2*pi
  Data Type Duplicate : DataTypeDuplicate
  Modulo : Math  Operator=mod  SaturateOnIntegerOverflow=on
  Sign1 : Signum
  Switch : Switch
  Angle_Flip : Outport
  wires:
  Switch/1 -> Data Type Duplicate/2, Angle_Flip/1
  Bias/1 -> Switch/3
  Sign1/1 -> Switch/2
  Modulo/1 -> Switch/1, Bias/1
  Constant/1 -> Modulo/2
  Angle/1 -> Data Type Duplicate/1, Sign1/1, Modulo/1
